simulink model "levitador_mpc_ss_du_restricoes_relaxamento"  (Simulink 7.9)
settings: Solver=ode5  SolverMode=SingleTasking  StartTime=0.0  StopTime=1  FixedStep=0.001  RelTol=1e-3
StartFcn:
  | disp('Início da simulação.')
  | clc
values from neighbouring files (symbols this model uses):
  Alp = [IM zeroM zeroM ... (first row only)    [matrizes_ss_du_restricoes_relaxamento.m]
  Aqp = [eye(M);-eye(M);TM;-TM;G;-G]    [matrizes_ss_du_restricoes_relaxamento.m]
  flp = [zeroM;d1;d2]    [matrizes_ss_du_restricoes_relaxamento.m]
  G = aux(:,1:M)    [matrizes_ss_du_restricoes_relaxamento.m]
  Hqp = 2*(G'*G + rho*eye(M))    [matrizes_ss_du_restricoes_relaxamento.m]
  r = yref*ones(N,1)    [mpc_ss_du_restricoes_relaxamento.m]
undefined symbols (not defined in the file or in its folder): A, B, C, dend, g, gamma, i0, Kf, mass, numd, Phi, T, up_equilibrio, y0, yp_equilibrio
settings Model: Creator=Kawakami  LastModifiedBy=Kawakami
settings DataIOCC: SignalLoggingName=sigsOut
settings OptimizationCC: BooleanDataType=off
settings DebuggingCC: SaveWithParameterizedLinksMsg=none  SignalResolutionControl=TryResolveAllWithWarning  SolverPrmCheckMsg=none  MultiTaskDSMMsg=warning  MultiTaskCondExecSysMsg=none  FcnCallInpInsideContextMsg=Use local settings  StrictBusMsg=None
settings HardwareCC: TargetUnknown=on
settings RTWCC: IncludeERTFirstTime=on
settings GRTTargetCC: CombineOutputUpdateFcns=off  GRTInterface=on

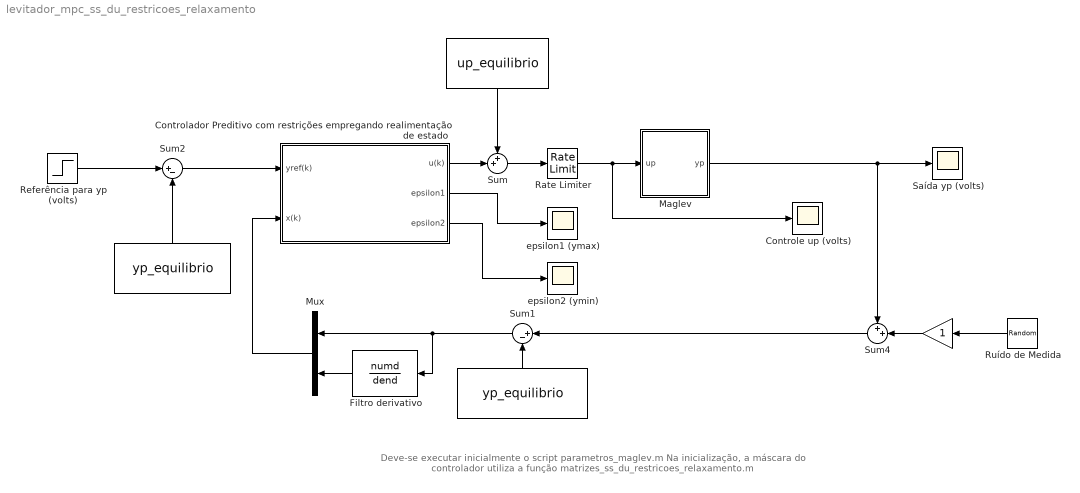
== system levitador_mpc_ss_du_restricoes_relaxamento ==
  note: Deve-se executar inicialmente o script parametros_maglev.m
      |
      | Na inicialização, a máscara do controlador utiliza a função matrizes_ss_du_restricoes_relaxamento.m
  " " : Constant  Value=yp_equilibrio
  "  " : Constant  Value=yp_equilibrio
  "   " : Constant  Value=up_equilibrio
  "     " : Gain
  Controlador Preditivo com restrições empregando realimentação de estado : Subsystem  mask{rho=1, N=10, M=5, A=A, B=B, C=C, up_equilibrio=up_equilibrio, yp_equilibrio=yp_equilibrio, dulim=[-0.25, 0.25], uplim=[-inf, inf], yplim=[-0.06 0.06], yplim_physical=[-inf, inf], d1=1, d2=1, relaxation_flag=1, T=T}
      mask prompts: rho "Peso do controle (rho)"; N "Horizonte de Predição (N)"; M "Horizonte de Controle (M)"; A "Matriz A"; B "Matriz B"; C "Matriz C"; dulim "[dumin, dumax]"; uplim "[upmin, upmax]"; yplim "[ypmin, ypmax]"; yplim_physical "[ypmin_physical,ypmax_physical]"; d1 "Peso da variável de folga associada a ymax (d1)"; d2 "Peso da variável de folga associada a ymin (d2)"; relaxation_flag "Usar relaxacao ? (0 = NAO, 1 = SIM)"; T "Periodo de amostragem"
      mask init:
      | [Phi,G,Hqp,Aqp,flp,Alp] = matrizes_ss_du_restricoes_relaxamento(A,B,C,N,M,rho,d1,d2);
      | ulim = uplim - up_equilibrio;
      | ylim = yplim - yp_equilibrio;
      | ylim_physical = yplim_physical - yp_equilibrio;
      | umin = ulim(1);
      | umax = ulim(2);
      | dumin = dulim(1);
      | dumax = dulim(2);
      | ymin = ylim(1);
      | ymax = ylim(2);
      | ymin_physical = ylim_physical(1);
      | ymax_physical = ylim_physical(2);
  Controle up (volts) : Scope
      settings: TimeRange=1  YMin=2.1  YMax=3.1  SaveName=y1
  Filtro derivativo : DiscreteTransferFcn  Numerator=numd  Denominator=dend  SampleTime=T
  Maglev : Subsystem  mask{mass=mass, g=g, y0=y0, gamma=gamma, i0=i0, r=r, Kf=Kf, y_inicial=yp_equilibrio, T=T}
      mask prompts: mass "mass (kg)"; g "g (m/s^2)"; y0 "y0 (V)"; gamma "gamma (V/m)"; i0 "i0 (A)"; r "r (A/V)"; Kf "Kf (N*m^2/A^2)"; y_inicial "y inicial (V)"; T "Periodo de Amostragem (s)"
  Mux : Mux  Inputs=2
  Rate Limiter : RateLimiter  RisingSlewLimit=0.25/T  FallingSlewLimit=-0.25/T
  Referência para yp (volts) : Step  Time=0  After=0  SampleTime=0
  Ruído de Medida : RandomNumber  Variance=0.0001  SampleTime=0
  Saída yp (volts) : Scope
      settings: TimeRange=1  YMin=-0.06  YMax=0.04000000000000001  SaveName=y
  Sum : Sum  Inputs=++|  SaturateOnIntegerOverflow=on
  Sum1 : Sum  Inputs=|+-  SaturateOnIntegerOverflow=on
  Sum2 : Sum  Inputs=|+-  SaturateOnIntegerOverflow=on
  Sum4 : Sum  Inputs=++|  SaturateOnIntegerOverflow=on
  epsilon1 (ymax) : Scope
      settings: TimeRange=1  YMin=-0.02  YMax=0.12  SaveName=y2
  epsilon2 (ymin) : Scope
      settings: TimeRange=1  YMin=-0.02  YMax=0.12  SaveName=y3
  wires:
  Controlador Preditivo com restrições empregando realimentação de estado/1(u(k)) -> Sum/2
  Sum2/1 -> Controlador Preditivo com restrições empregando realimentação de estado/1(yref(k))
  Referência para yp (volts)/1 -> Sum2/1
  Maglev/1(yp) -> Saída yp (volts)/1, Sum4/1
  Sum4/1 -> Sum1/1
  Sum/1 -> Rate Limiter/1
  " "/1 -> Sum1/2
  "  "/1 -> Sum2/2
  "   "/1 -> Sum/1
  Ruído de Medida/1 -> "     "/1
  Sum1/1 -> Mux/1, Filtro derivativo/1
  Mux/1 -> Controlador Preditivo com restrições empregando realimentação de estado/2(x(k))
  Filtro derivativo/1 -> Mux/2
  Rate Limiter/1 -> Controle up (volts)/1, Maglev/1(up)
  Controlador Preditivo com restrições empregando realimentação de estado/2(epsilon1) -> epsilon1 (ymax)/1
  Controlador Preditivo com restrições empregando realimentação de estado/3(epsilon2) -> epsilon2 (ymin)/1
  "     "/1 -> Sum4/2

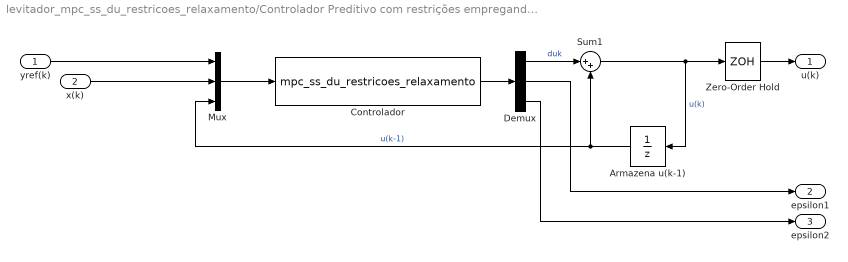
== system levitador_mpc_ss_du_restricoes_relaxamento/Controlador Preditivo com restrições empregando realimentação de estado ==
  yref(k) : Inport
  x(k) : Inport  Port=2
  Armazena u(k-1) : UnitDelay  SampleTime=T
  Controlador : S-Function  FunctionName=mpc_ss_du_restricoes_relaxamento  Parameters=Phi,G,Hqp,Aqp,flp,Alp,dumax,dumin,umax,umin,ymax,ymin,ymax_physical,ymin_physical,M,N,relaxation_flag,T  EnableBusSupport=off
  Demux : Demux  Outputs=3
  Mux : Mux  Inputs=3
  Sum1 : Sum  Inputs=|++  SaturateOnIntegerOverflow=on  InputSameDT=on  OutDataTypeStr=Inherit: Same as first input
  Zero-Order Hold : ZeroOrderHold  SampleTime=T
  u(k) : Outport
  epsilon1 : Outport  Port=2
  epsilon2 : Outport  Port=3
  wires:
  Mux/1 -> Controlador/1
  Zero-Order Hold/1 -> u(k)/1
  x(k)/1 -> Mux/2
  yref(k)/1 -> Mux/1
  Sum1/1 -> Zero-Order Hold/1, Armazena u(k-1)/1  "u(k)"
  Armazena u(k-1)/1 -> Sum1/2, Mux/3  "u(k-1)"
  Controlador/1 -> Demux/1
  Demux/1 -> Sum1/1  "duk"
  Demux/3 -> epsilon2/1
  Demux/2 -> epsilon1/1

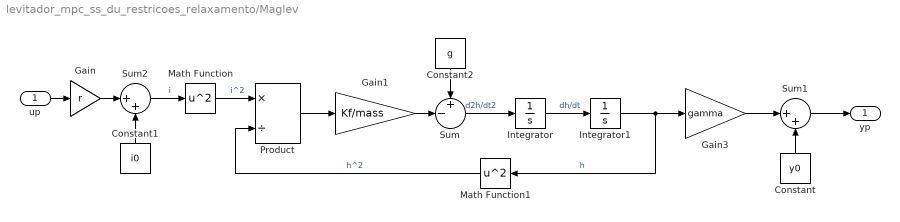
== system levitador_mpc_ss_du_restricoes_relaxamento/Maglev ==
  up : Inport
  Constant : Constant  Value=y0
  Constant1 : Constant  Value=i0
  Constant2 : Constant  Value=g
  Gain : Gain  Gain=r  SaturateOnIntegerOverflow=on  OutDataTypeStr=Inherit: Same as input  ParamDataTypeStr=Inherit: Same as input
  Gain1 : Gain  Gain=Kf/mass  SaturateOnIntegerOverflow=on  OutDataTypeStr=Inherit: Same as input  ParamDataTypeStr=Inherit: Same as input
  Gain3 : Gain  Gain=gamma  SaturateOnIntegerOverflow=on  OutDataTypeStr=Inherit: Same as input  ParamDataTypeStr=Inherit: Same as input
  Integrator : Integrator
  Integrator1 : Integrator  InitialCondition=(y_inicial - y0)/gamma
  Math Function : Math  Operator=square  SaturateOnIntegerOverflow=on
  Math Function1 : Math  Operator=square  SaturateOnIntegerOverflow=on
  Product : Product  Inputs=*/  SaturateOnIntegerOverflow=on  OutDataTypeStr=Inherit: Same as first input
  Sum : Sum  Inputs=+-|  SaturateOnIntegerOverflow=on
  Sum1 : Sum  Inputs=|++  SaturateOnIntegerOverflow=on
  Sum2 : Sum  Inputs=|++  SaturateOnIntegerOverflow=on
  yp : Outport
  wires:
  Integrator/1 -> Integrator1/1  "dh/dt"
  Sum/1 -> Integrator/1  "d2h/dt2"
  Integrator1/1 -> Gain3/1, Math Function1/1  "h"
  up/1 -> Gain/1
  Constant/1 -> Sum1/2
  Gain3/1 -> Sum1/1
  Sum1/1 -> yp/1
  Constant1/1 -> Sum2/2
  Gain/1 -> Sum2/1
  Sum2/1 -> Math Function/1  "i"
  Math Function/1 -> Product/1  "i^2"
  Math Function1/1 -> Product/2  "h^2"
  Product/1 -> Gain1/1
  Gain1/1 -> Sum/2
  Constant2/1 -> Sum/1
